simulink library "INT_DrvDem_CalcState"  (R2016b)
settings: Solver=VariableStepAuto  StartTime=0.0  StopTime=10.0  RelTol=1e-3
settings Model: Creator=xuxingpei  LastModifiedBy=xuxingpei

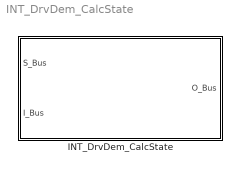
== system INT_DrvDem_CalcState ==
  INT_DrvDem_CalcState : Subsystem

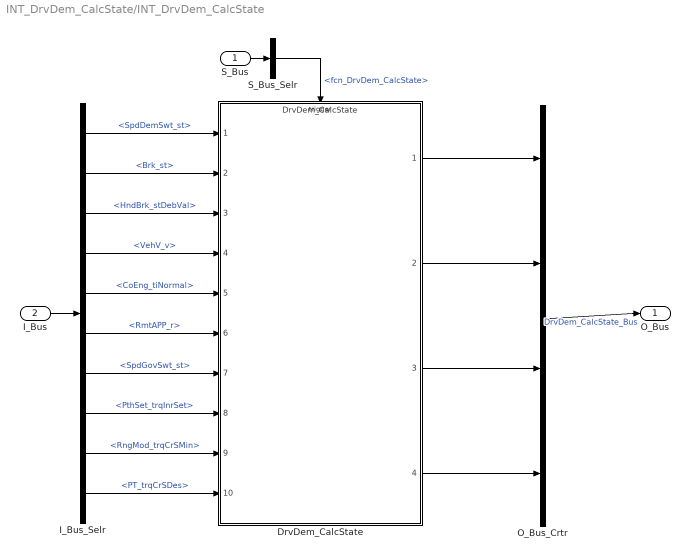
== system INT_DrvDem_CalcState/INT_DrvDem_CalcState ==
  S_Bus : Inport
  I_Bus : Inport  Port=2
  DrvDem_CalcState : ModelReference  ModelNameDialog=DrvDem_CalcState  SimulationMode=Normal  ModelReferenceVersion=1.66  TriggerPortName=function  TriggerPortTriggerType=function-call  TriggerPortStatesWhenEnabling=held
  I_Bus_Selr : BusSelector  OutputSignals=SpdDemSwt_st,Brk_st,HndBrk_stDebVal,VehV_v,CoEng_tiNormal,RmtAPP_r,SpdGovSwt_st,PthSet_trqInrSet,RngMod_trqCrSMin,PT_trqCrSDes
  O_Bus_Crtr : BusCreator  Inputs=4
  S_Bus_Selr : BusSelector  OutputSignals=fcn_DrvDem_CalcState
  O_Bus : Outport
  wires:
  S_Bus_Selr/1 -> DrvDem_CalcState/Trigger  "<fcn_DrvDem_CalcState>"
  S_Bus/1 -> S_Bus_Selr/1
  I_Bus/1 -> I_Bus_Selr/1
  I_Bus_Selr/1 -> DrvDem_CalcState/1  "<SpdDemSwt_st>"
  I_Bus_Selr/2 -> DrvDem_CalcState/2  "<Brk_st>"
  I_Bus_Selr/3 -> DrvDem_CalcState/3  "<HndBrk_stDebVal>"
  I_Bus_Selr/4 -> DrvDem_CalcState/4  "<VehV_v>"
  I_Bus_Selr/5 -> DrvDem_CalcState/5  "<CoEng_tiNormal>"
  I_Bus_Selr/6 -> DrvDem_CalcState/6  "<RmtAPP_r>"
  I_Bus_Selr/7 -> DrvDem_CalcState/7  "<SpdGovSwt_st>"
  I_Bus_Selr/8 -> DrvDem_CalcState/8  "<PthSet_trqInrSet>"
  I_Bus_Selr/9 -> DrvDem_CalcState/9  "<RngMod_trqCrSMin>"
  I_Bus_Selr/10 -> DrvDem_CalcState/10  "<PT_trqCrSDes>"
  O_Bus_Crtr/1 -> O_Bus/1  "DrvDem_CalcState_Bus"
  DrvDem_CalcState/1 -> O_Bus_Crtr/1
  DrvDem_CalcState/2 -> O_Bus_Crtr/2
  DrvDem_CalcState/3 -> O_Bus_Crtr/3
  DrvDem_CalcState/4 -> O_Bus_Crtr/4
